simulink model "stewart_platform"  (R2013a)
settings: Solver=ode45  StartTime=0.0  StopTime=10.0  RelTol=1e-3
undefined symbols (not defined in the file): X, Y, Z
libraries: sm_lib x1374, nesl_utility x1
(part 29 of 30)

== system stewart_platform/BaseRingAssembly_1_RIGID/SwivelBearing3_1_RIGID/swivelbearingshaft_1_RIGID/Yoke_1_RIGID ==
  ReferenceFrame : sm_lib/Frames and  Transforms/Reference  Frame  BlockFunction=simmechanics.library.frames_transforms.reference_frame
  Solid : sm_lib/Body Elements/Solid  InertiaType=Custom  Mass=0.0085668099999999994  MassUnits=kg  CenterOfMass=[3.3036099999999999e-09 4.5392100000000001e-09 0.0138091]  CenterOfMassUnits=m  MomentsOfInertia=[3.6198600000000002e-07 3.7260700000000002e-07 1.1777300000000001e-07]  MomentsOfInertiaUnits=kg*m^2  ProductsOfInertia=[-1.58919e-13 -3.9281799999999999e-13 1.96468e-13]  ProductsOfInertiaUnits=kg*m^2  DensityBased=on  Density=1000  DensityUnits=kg/(m^3)  GraphicType=FromGeometry  MarkerShape=Sphere  MarkerSize=10  MarkerSizeUnits=m  GraphicVisPropType=SimpleVisualProperties  GraphicDiffuseColor=[0.594824 0.594824 0.594824]  GraphicSpecularColor=[0.5 0.5 0.5 1.0]  GraphicAmbientColor=[0.15 0.15 0.15 1.0]  GraphicEmissiveColor=[0.0 0.0 0.0 1.0]  GraphicShininess=75  GraphicOpacity=1  GeometryShape=FromFile  RectangleSize=[1 1]  RectangleSizeUnits=m  BrickDimensions=[1 1 1]  BrickDimensionUnits=m  CylinderRadius=1  CylinderRadiusUnits=m  CylinderLength=1  CylinderLengthUnits=m  SphereRadius=1  SphereRadiusUnits=m  EllipsoidRadii=[1 1 1]  EllipsoidRadiiUnits=m  ExtrusionCrossSection=[1 1; -1 1; -1 -1; 1 -1]  ExtrusionCrossSectionUnits=m  ExtrusionLength=1  ExtrusionLengthUnits=m  PolygonNumSides=3  PolygonOuterRadius=1  PolygonOuterRadiusUnits=m  ExtGeomFileName=Yoke_Default_sldprt.STL  ExtGeomFileUnits=m  RevolutionCrossSection=[1 1; 1 -1; 2 -1; 2 1]  RevolutionCrossSectionUnits=m  RevolutionExtent=Full  RevolutionAngle=180  RevolutionAngleUnits=deg  BlockFunction=simmechanics.library.body_elements.solid
  F : PMIOPort  Port=1  Side=Left
  connections:
  Solid/RConn1 -- ReferenceFrame/RConn1 -- F/RConn1

== system stewart_platform/BaseRingAssembly_1_RIGID/SwivelBearing4_1_RIGID/swivelbearingbase_1_RIGID/Bearing_Block_1_RIGID ==
  ReferenceFrame : sm_lib/Frames and  Transforms/Reference  Frame  BlockFunction=simmechanics.library.frames_transforms.reference_frame
  Solid : sm_lib/Body Elements/Solid  InertiaType=Custom  Mass=0.038815299999999997  MassUnits=kg  CenterOfMass=[1.2331699999999999 -2.0896699999999997e-06 -0.091549200000000011]  CenterOfMassUnits=cm  MomentsOfInertia=[0.037792699999999999 0.030256599999999998 0.030404499999999998]  MomentsOfInertiaUnits=kg*cm^2  ProductsOfInertia=[2.5125199999999998e-07 -0.0029988099999999998 -2.7532300000000001e-08]  ProductsOfInertiaUnits=kg*cm^2  DensityBased=on  Density=1000  DensityUnits=kg/(m^3)  GraphicType=FromGeometry  MarkerShape=Sphere  MarkerSize=10  MarkerSizeUnits=m  GraphicVisPropType=SimpleVisualProperties  GraphicDiffuseColor=[0.308706 0.308706 0.308706]  GraphicSpecularColor=[0.5 0.5 0.5 1.0]  GraphicAmbientColor=[0.15 0.15 0.15 1.0]  GraphicEmissiveColor=[0.0 0.0 0.0 1.0]  GraphicShininess=75  GraphicOpacity=1  GeometryShape=FromFile  RectangleSize=[1 1]  RectangleSizeUnits=m  BrickDimensions=[1 1 1]  BrickDimensionUnits=m  CylinderRadius=1  CylinderRadiusUnits=m  CylinderLength=1  CylinderLengthUnits=m  SphereRadius=1  SphereRadiusUnits=m  EllipsoidRadii=[1 1 1]  EllipsoidRadiiUnits=m  ExtrusionCrossSection=[1 1; -1 1; -1 -1; 1 -1]  ExtrusionCrossSectionUnits=m  ExtrusionLength=1  ExtrusionLengthUnits=m  PolygonNumSides=3  PolygonOuterRadius=1  PolygonOuterRadiusUnits=m  ExtGeomFileName=Bearing_Block_Default_sldprt.STL  ExtGeomFileUnits=cm  RevolutionCrossSection=[1 1; 1 -1; 2 -1; 2 1]  RevolutionCrossSectionUnits=m  RevolutionExtent=Full  RevolutionAngle=180  RevolutionAngleUnits=deg  BlockFunction=simmechanics.library.body_elements.solid
  F : PMIOPort  Port=1  Side=Left
  connections:
  Solid/RConn1 -- ReferenceFrame/RConn1 -- F/RConn1

== system stewart_platform/BaseRingAssembly_1_RIGID/SwivelBearing4_1_RIGID/swivelbearingbase_1_RIGID/Clevis_pin_A_3x6_1_RIGID ==
  ReferenceFrame : sm_lib/Frames and  Transforms/Reference  Frame  BlockFunction=simmechanics.library.frames_transforms.reference_frame
  Solid : sm_lib/Body Elements/Solid  InertiaType=Custom  Mass=0.00029381199999999996  MassUnits=kg  CenterOfMass=[0.29999999999999999 0 0]  CenterOfMassUnits=cm  MomentsOfInertia=[3.0689199999999997e-06 8.8308599999999993e-06 8.8308599999999993e-06]  MomentsOfInertiaUnits=kg*cm^2  ProductsOfInertia=[0 0 0]  ProductsOfInertiaUnits=kg*cm^2  DensityBased=on  Density=1000  DensityUnits=kg/(m^3)  GraphicType=FromGeometry  MarkerShape=Sphere  MarkerSize=10  MarkerSizeUnits=m  GraphicVisPropType=SimpleVisualProperties  GraphicDiffuseColor=[0.594824 0.594824 0.594824]  GraphicSpecularColor=[0.5 0.5 0.5 1.0]  GraphicAmbientColor=[0.15 0.15 0.15 1.0]  GraphicEmissiveColor=[0.0 0.0 0.0 1.0]  GraphicShininess=75  GraphicOpacity=1  GeometryShape=FromFile  RectangleSize=[1 1]  RectangleSizeUnits=m  BrickDimensions=[1 1 1]  BrickDimensionUnits=m  CylinderRadius=1  CylinderRadiusUnits=m  CylinderLength=1  CylinderLengthUnits=m  SphereRadius=1  SphereRadiusUnits=m  EllipsoidRadii=[1 1 1]  EllipsoidRadiiUnits=m  ExtrusionCrossSection=[1 1; -1 1; -1 -1; 1 -1]  ExtrusionCrossSectionUnits=m  ExtrusionLength=1  ExtrusionLengthUnits=m  PolygonNumSides=3  PolygonOuterRadius=1  PolygonOuterRadiusUnits=m  ExtGeomFileName=Clevis_pin_A_3x6_Default_sldprt.STL  ExtGeomFileUnits=cm  RevolutionCrossSection=[1 1; 1 -1; 2 -1; 2 1]  RevolutionCrossSectionUnits=m  RevolutionExtent=Full  RevolutionAngle=180  RevolutionAngleUnits=deg  BlockFunction=simmechanics.library.body_elements.solid
  F : PMIOPort  Port=1  Side=Left
  connections:
  Solid/RConn1 -- ReferenceFrame/RConn1 -- F/RConn1

== system stewart_platform/BaseRingAssembly_1_RIGID/SwivelBearing4_1_RIGID/swivelbearingbase_1_RIGID/Clevis_pin_A_3x6_2_RIGID ==
  ReferenceFrame : sm_lib/Frames and  Transforms/Reference  Frame  BlockFunction=simmechanics.library.frames_transforms.reference_frame
  Solid : sm_lib/Body Elements/Solid  InertiaType=Custom  Mass=0.00029381199999999996  MassUnits=kg  CenterOfMass=[0.29999999999999999 0 0]  CenterOfMassUnits=cm  MomentsOfInertia=[3.0689199999999997e-06 8.8308599999999993e-06 8.8308599999999993e-06]  MomentsOfInertiaUnits=kg*cm^2  ProductsOfInertia=[0 0 0]  ProductsOfInertiaUnits=kg*cm^2  DensityBased=on  Density=1000  DensityUnits=kg/(m^3)  GraphicType=FromGeometry  MarkerShape=Sphere  MarkerSize=10  MarkerSizeUnits=m  GraphicVisPropType=SimpleVisualProperties  GraphicDiffuseColor=[0.594824 0.594824 0.594824]  GraphicSpecularColor=[0.5 0.5 0.5 1.0]  GraphicAmbientColor=[0.15 0.15 0.15 1.0]  GraphicEmissiveColor=[0.0 0.0 0.0 1.0]  GraphicShininess=75  GraphicOpacity=1  GeometryShape=FromFile  RectangleSize=[1 1]  RectangleSizeUnits=m  BrickDimensions=[1 1 1]  BrickDimensionUnits=m  CylinderRadius=1  CylinderRadiusUnits=m  CylinderLength=1  CylinderLengthUnits=m  SphereRadius=1  SphereRadiusUnits=m  EllipsoidRadii=[1 1 1]  EllipsoidRadiiUnits=m  ExtrusionCrossSection=[1 1; -1 1; -1 -1; 1 -1]  ExtrusionCrossSectionUnits=m  ExtrusionLength=1  ExtrusionLengthUnits=m  PolygonNumSides=3  PolygonOuterRadius=1  PolygonOuterRadiusUnits=m  ExtGeomFileName=Clevis_pin_A_3x6_Default_sldprt.STL  ExtGeomFileUnits=cm  RevolutionCrossSection=[1 1; 1 -1; 2 -1; 2 1]  RevolutionCrossSectionUnits=m  RevolutionExtent=Full  RevolutionAngle=180  RevolutionAngleUnits=deg  BlockFunction=simmechanics.library.body_elements.solid
  F : PMIOPort  Port=1  Side=Left
  connections:
  Solid/RConn1 -- ReferenceFrame/RConn1 -- F/RConn1

== system stewart_platform/BaseRingAssembly_1_RIGID/SwivelBearing4_1_RIGID/swivelbearingbase_1_RIGID/Cylinder_Head_Cap_Screw_M3x10_1_RIGID ==
  ReferenceFrame : sm_lib/Frames and  Transforms/Reference  Frame  BlockFunction=simmechanics.library.frames_transforms.reference_frame
  Solid : sm_lib/Body Elements/Solid  InertiaType=Custom  Mass=0.00086707500000000014  MassUnits=kg  CenterOfMass=[0.27793600000000002 4.4415200000000001e-05 3.1751399999999999e-07]  CenterOfMassUnits=cm  MomentsOfInertia=[1.96811e-05 0.000127587 0.000127572]  MomentsOfInertiaUnits=kg*cm^2  ProductsOfInertia=[9.9546899999999997e-10 -9.8543100000000009e-11 -1.3784599999999999e-08]  ProductsOfInertiaUnits=kg*cm^2  DensityBased=on  Density=1000  DensityUnits=kg/(m^3)  GraphicType=FromGeometry  MarkerShape=Sphere  MarkerSize=10  MarkerSizeUnits=m  GraphicVisPropType=SimpleVisualProperties  GraphicDiffuseColor=[0.722824 0.722824 0.722824]  GraphicSpecularColor=[0.5 0.5 0.5 1.0]  GraphicAmbientColor=[0.15 0.15 0.15 1.0]  GraphicEmissiveColor=[0.0 0.0 0.0 1.0]  GraphicShininess=75  GraphicOpacity=1  GeometryShape=FromFile  RectangleSize=[1 1]  RectangleSizeUnits=m  BrickDimensions=[1 1 1]  BrickDimensionUnits=m  CylinderRadius=1  CylinderRadiusUnits=m  CylinderLength=1  CylinderLengthUnits=m  SphereRadius=1  SphereRadiusUnits=m  EllipsoidRadii=[1 1 1]  EllipsoidRadiiUnits=m  ExtrusionCrossSection=[1 1; -1 1; -1 -1; 1 -1]  ExtrusionCrossSectionUnits=m  ExtrusionLength=1  ExtrusionLengthUnits=m  PolygonNumSides=3  PolygonOuterRadius=1  PolygonOuterRadiusUnits=m  ExtGeomFileName=Cylinder_Head_Cap_Screw_M3x10_Default_sldprt.STL  ExtGeomFileUnits=cm  RevolutionCrossSection=[1 1; 1 -1; 2 -1; 2 1]  RevolutionCrossSectionUnits=m  RevolutionExtent=Full  RevolutionAngle=180  RevolutionAngleUnits=deg  BlockFunction=simmechanics.library.body_elements.solid
  F : PMIOPort  Port=1  Side=Left
  connections:
  Solid/RConn1 -- ReferenceFrame/RConn1 -- F/RConn1

== system stewart_platform/BaseRingAssembly_1_RIGID/SwivelBearing4_1_RIGID/swivelbearingbase_1_RIGID/Cylinder_Head_Cap_Screw_M3x10_2_RIGID ==
  ReferenceFrame : sm_lib/Frames and  Transforms/Reference  Frame  BlockFunction=simmechanics.library.frames_transforms.reference_frame
  Solid : sm_lib/Body Elements/Solid  InertiaType=Custom  Mass=0.00086707500000000014  MassUnits=kg  CenterOfMass=[0.27793600000000002 4.4415200000000001e-05 3.1751399999999999e-07]  CenterOfMassUnits=cm  MomentsOfInertia=[1.96811e-05 0.000127587 0.000127572]  MomentsOfInertiaUnits=kg*cm^2  ProductsOfInertia=[9.9546899999999997e-10 -9.8543100000000009e-11 -1.3784599999999999e-08]  ProductsOfInertiaUnits=kg*cm^2  DensityBased=on  Density=1000  DensityUnits=kg/(m^3)  GraphicType=FromGeometry  MarkerShape=Sphere  MarkerSize=10  MarkerSizeUnits=m  GraphicVisPropType=SimpleVisualProperties  GraphicDiffuseColor=[0.722824 0.722824 0.722824]  GraphicSpecularColor=[0.5 0.5 0.5 1.0]  GraphicAmbientColor=[0.15 0.15 0.15 1.0]  GraphicEmissiveColor=[0.0 0.0 0.0 1.0]  GraphicShininess=75  GraphicOpacity=1  GeometryShape=FromFile  RectangleSize=[1 1]  RectangleSizeUnits=m  BrickDimensions=[1 1 1]  BrickDimensionUnits=m  CylinderRadius=1  CylinderRadiusUnits=m  CylinderLength=1  CylinderLengthUnits=m  SphereRadius=1  SphereRadiusUnits=m  EllipsoidRadii=[1 1 1]  EllipsoidRadiiUnits=m  ExtrusionCrossSection=[1 1; -1 1; -1 -1; 1 -1]  ExtrusionCrossSectionUnits=m  ExtrusionLength=1  ExtrusionLengthUnits=m  PolygonNumSides=3  PolygonOuterRadius=1  PolygonOuterRadiusUnits=m  ExtGeomFileName=Cylinder_Head_Cap_Screw_M3x10_Default_sldprt.STL  ExtGeomFileUnits=cm  RevolutionCrossSection=[1 1; 1 -1; 2 -1; 2 1]  RevolutionCrossSectionUnits=m  RevolutionExtent=Full  RevolutionAngle=180  RevolutionAngleUnits=deg  BlockFunction=simmechanics.library.body_elements.solid
  F : PMIOPort  Port=1  Side=Left
  connections:
  Solid/RConn1 -- ReferenceFrame/RConn1 -- F/RConn1

== system stewart_platform/BaseRingAssembly_1_RIGID/SwivelBearing4_1_RIGID/swivelbearingbase_1_RIGID/MPB_C345MB_1_RIGID ==
  ReferenceFrame : sm_lib/Frames and  Transforms/Reference  Frame  BlockFunction=simmechanics.library.frames_transforms.reference_frame
  Solid : sm_lib/Body Elements/Solid  InertiaType=Custom  Mass=0.0062849100000000003  MassUnits=kg  CenterOfMass=[-0.00467958 0.00015178199999999999 0]  CenterOfMassUnits=cm  MomentsOfInertia=[0.0022913899999999999 0.0012611399999999998 0.0012599700000000002]  MomentsOfInertiaUnits=kg*cm^2  ProductsOfInertia=[0 8.7957900000000007e-09 4.4951200000000001e-09]  ProductsOfInertiaUnits=kg*cm^2  DensityBased=on  Density=1000  DensityUnits=kg/(m^3)  GraphicType=FromGeometry  MarkerShape=Sphere  MarkerSize=10  MarkerSizeUnits=m  GraphicVisPropType=SimpleVisualProperties  GraphicDiffuseColor=[0.722824 0.722824 0.722824]  GraphicSpecularColor=[0.5 0.5 0.5 1.0]  GraphicAmbientColor=[0.15 0.15 0.15 1.0]  GraphicEmissiveColor=[0.0 0.0 0.0 1.0]  GraphicShininess=75  GraphicOpacity=1  GeometryShape=FromFile  RectangleSize=[1 1]  RectangleSizeUnits=m  BrickDimensions=[1 1 1]  BrickDimensionUnits=m  CylinderRadius=1  CylinderRadiusUnits=m  CylinderLength=1  CylinderLengthUnits=m  SphereRadius=1  SphereRadiusUnits=m  EllipsoidRadii=[1 1 1]  EllipsoidRadiiUnits=m  ExtrusionCrossSection=[1 1; -1 1; -1 -1; 1 -1]  ExtrusionCrossSectionUnits=m  ExtrusionLength=1  ExtrusionLengthUnits=m  PolygonNumSides=3  PolygonOuterRadius=1  PolygonOuterRadiusUnits=m  ExtGeomFileName=MPB_C345MB_Default_sldprt.STL  ExtGeomFileUnits=cm  RevolutionCrossSection=[1 1; 1 -1; 2 -1; 2 1]  RevolutionCrossSectionUnits=m  RevolutionExtent=Full  RevolutionAngle=180  RevolutionAngleUnits=deg  BlockFunction=simmechanics.library.body_elements.solid
  F : PMIOPort  Port=1  Side=Left
  connections:
  Solid/RConn1 -- ReferenceFrame/RConn1 -- F/RConn1

== system stewart_platform/BaseRingAssembly_1_RIGID/SwivelBearing4_1_RIGID/swivelbearingbase_1_RIGID/MPB_C345MB_2_RIGID ==
  ReferenceFrame : sm_lib/Frames and  Transforms/Reference  Frame  BlockFunction=simmechanics.library.frames_transforms.reference_frame
  Solid : sm_lib/Body Elements/Solid  InertiaType=Custom  Mass=0.0062849100000000003  MassUnits=kg  CenterOfMass=[-0.00467958 0.00015178199999999999 0]  CenterOfMassUnits=cm  MomentsOfInertia=[0.0022913899999999999 0.0012611399999999998 0.0012599700000000002]  MomentsOfInertiaUnits=kg*cm^2  ProductsOfInertia=[0 8.7957900000000007e-09 4.4951200000000001e-09]  ProductsOfInertiaUnits=kg*cm^2  DensityBased=on  Density=1000  DensityUnits=kg/(m^3)  GraphicType=FromGeometry  MarkerShape=Sphere  MarkerSize=10  MarkerSizeUnits=m  GraphicVisPropType=SimpleVisualProperties  GraphicDiffuseColor=[0.722824 0.722824 0.722824]  GraphicSpecularColor=[0.5 0.5 0.5 1.0]  GraphicAmbientColor=[0.15 0.15 0.15 1.0]  GraphicEmissiveColor=[0.0 0.0 0.0 1.0]  GraphicShininess=75  GraphicOpacity=1  GeometryShape=FromFile  RectangleSize=[1 1]  RectangleSizeUnits=m  BrickDimensions=[1 1 1]  BrickDimensionUnits=m  CylinderRadius=1  CylinderRadiusUnits=m  CylinderLength=1  CylinderLengthUnits=m  SphereRadius=1  SphereRadiusUnits=m  EllipsoidRadii=[1 1 1]  EllipsoidRadiiUnits=m  ExtrusionCrossSection=[1 1; -1 1; -1 -1; 1 -1]  ExtrusionCrossSectionUnits=m  ExtrusionLength=1  ExtrusionLengthUnits=m  PolygonNumSides=3  PolygonOuterRadius=1  PolygonOuterRadiusUnits=m  ExtGeomFileName=MPB_C345MB_Default_sldprt.STL  ExtGeomFileUnits=cm  RevolutionCrossSection=[1 1; 1 -1; 2 -1; 2 1]  RevolutionCrossSectionUnits=m  RevolutionExtent=Full  RevolutionAngle=180  RevolutionAngleUnits=deg  BlockFunction=simmechanics.library.body_elements.solid
  F : PMIOPort  Port=1  Side=Left
  connections:
  Solid/RConn1 -- ReferenceFrame/RConn1 -- F/RConn1

== system stewart_platform/BaseRingAssembly_1_RIGID/SwivelBearing4_1_RIGID/swivelbearingshaft_1_RIGID/Hex_Nut_M5_1_RIGID ==
  ReferenceFrame : sm_lib/Frames and  Transforms/Reference  Frame  BlockFunction=simmechanics.library.frames_transforms.reference_frame
  Solid : sm_lib/Body Elements/Solid  InertiaType=Custom  Mass=0.0014621200000000001  MassUnits=kg  CenterOfMass=[0.23500000000000001 8.4057099999999999e-13 -1.6260300000000001e-12]  CenterOfMassUnits=cm  MomentsOfInertia=[0.00015881600000000002 0.000103959 0.00010395999999999999]  MomentsOfInertiaUnits=kg*cm^2  ProductsOfInertia=[-1.13877e-10 -2.0700200000000003e-10 0]  ProductsOfInertiaUnits=kg*cm^2  DensityBased=on  Density=1000  DensityUnits=kg/(m^3)  GraphicType=FromGeometry  MarkerShape=Sphere  MarkerSize=10  MarkerSizeUnits=m  GraphicVisPropType=SimpleVisualProperties  GraphicDiffuseColor=[0.594824 0.594824 0.594824]  GraphicSpecularColor=[0.5 0.5 0.5 1.0]  GraphicAmbientColor=[0.15 0.15 0.15 1.0]  GraphicEmissiveColor=[0.0 0.0 0.0 1.0]  GraphicShininess=75  GraphicOpacity=1  GeometryShape=FromFile  RectangleSize=[1 1]  RectangleSizeUnits=m  BrickDimensions=[1 1 1]  BrickDimensionUnits=m  CylinderRadius=1  CylinderRadiusUnits=m  CylinderLength=1  CylinderLengthUnits=m  SphereRadius=1  SphereRadiusUnits=m  EllipsoidRadii=[1 1 1]  EllipsoidRadiiUnits=m  ExtrusionCrossSection=[1 1; -1 1; -1 -1; 1 -1]  ExtrusionCrossSectionUnits=m  ExtrusionLength=1  ExtrusionLengthUnits=m  PolygonNumSides=3  PolygonOuterRadius=1  PolygonOuterRadiusUnits=m  ExtGeomFileName=Hex_Nut_M5_Default_sldprt.STL  ExtGeomFileUnits=cm  RevolutionCrossSection=[1 1; 1 -1; 2 -1; 2 1]  RevolutionCrossSectionUnits=m  RevolutionExtent=Full  RevolutionAngle=180  RevolutionAngleUnits=deg  BlockFunction=simmechanics.library.body_elements.solid
  F : PMIOPort  Port=1  Side=Left
  connections:
  Solid/RConn1 -- ReferenceFrame/RConn1 -- F/RConn1

== system stewart_platform/BaseRingAssembly_1_RIGID/SwivelBearing4_1_RIGID/swivelbearingshaft_1_RIGID/Threaded_Shaft_1_RIGID ==
  ReferenceFrame : sm_lib/Frames and  Transforms/Reference  Frame  BlockFunction=simmechanics.library.frames_transforms.reference_frame
  Solid : sm_lib/Body Elements/Solid  InertiaType=Custom  Mass=0.006728679999999999  MassUnits=kg  CenterOfMass=[0 -1.6645400000000003e-08 2.24966]  CenterOfMassUnits=cm  MomentsOfInertia=[0.011498500000000002 0.011501300000000001 0.00020671399999999999]  MomentsOfInertiaUnits=kg*cm^2  ProductsOfInertia=[-1.35425e-10 0 0]  ProductsOfInertiaUnits=kg*cm^2  DensityBased=on  Density=1000  DensityUnits=kg/(m^3)  GraphicType=FromGeometry  MarkerShape=Sphere  MarkerSize=10  MarkerSizeUnits=m  GraphicVisPropType=SimpleVisualProperties  GraphicDiffuseColor=[0.594824 0.594824 0.594824]  GraphicSpecularColor=[0.5 0.5 0.5 1.0]  GraphicAmbientColor=[0.15 0.15 0.15 1.0]  GraphicEmissiveColor=[0.0 0.0 0.0 1.0]  GraphicShininess=75  GraphicOpacity=1  GeometryShape=FromFile  RectangleSize=[1 1]  RectangleSizeUnits=m  BrickDimensions=[1 1 1]  BrickDimensionUnits=m  CylinderRadius=1  CylinderRadiusUnits=m  CylinderLength=1  CylinderLengthUnits=m  SphereRadius=1  SphereRadiusUnits=m  EllipsoidRadii=[1 1 1]  EllipsoidRadiiUnits=m  ExtrusionCrossSection=[1 1; -1 1; -1 -1; 1 -1]  ExtrusionCrossSectionUnits=m  ExtrusionLength=1  ExtrusionLengthUnits=m  PolygonNumSides=3  PolygonOuterRadius=1  PolygonOuterRadiusUnits=m  ExtGeomFileName=Threaded_Shaft_Default_sldprt.STL  ExtGeomFileUnits=cm  RevolutionCrossSection=[1 1; 1 -1; 2 -1; 2 1]  RevolutionCrossSectionUnits=m  RevolutionExtent=Full  RevolutionAngle=180  RevolutionAngleUnits=deg  BlockFunction=simmechanics.library.body_elements.solid
  F : PMIOPort  Port=1  Side=Left
  connections:
  Solid/RConn1 -- ReferenceFrame/RConn1 -- F/RConn1

== system stewart_platform/BaseRingAssembly_1_RIGID/SwivelBearing4_1_RIGID/swivelbearingshaft_1_RIGID/Yoke_1_RIGID ==
  ReferenceFrame : sm_lib/Frames and  Transforms/Reference  Frame  BlockFunction=simmechanics.library.frames_transforms.reference_frame
  Solid : sm_lib/Body Elements/Solid  InertiaType=Custom  Mass=0.0085668099999999994  MassUnits=kg  CenterOfMass=[3.3036099999999999e-09 4.5392100000000001e-09 0.0138091]  CenterOfMassUnits=m  MomentsOfInertia=[3.6198600000000002e-07 3.7260700000000002e-07 1.1777300000000001e-07]  MomentsOfInertiaUnits=kg*m^2  ProductsOfInertia=[-1.58919e-13 -3.9281799999999999e-13 1.96468e-13]  ProductsOfInertiaUnits=kg*m^2  DensityBased=on  Density=1000  DensityUnits=kg/(m^3)  GraphicType=FromGeometry  MarkerShape=Sphere  MarkerSize=10  MarkerSizeUnits=m  GraphicVisPropType=SimpleVisualProperties  GraphicDiffuseColor=[0.594824 0.594824 0.594824]  GraphicSpecularColor=[0.5 0.5 0.5 1.0]  GraphicAmbientColor=[0.15 0.15 0.15 1.0]  GraphicEmissiveColor=[0.0 0.0 0.0 1.0]  GraphicShininess=75  GraphicOpacity=1  GeometryShape=FromFile  RectangleSize=[1 1]  RectangleSizeUnits=m  BrickDimensions=[1 1 1]  BrickDimensionUnits=m  CylinderRadius=1  CylinderRadiusUnits=m  CylinderLength=1  CylinderLengthUnits=m  SphereRadius=1  SphereRadiusUnits=m  EllipsoidRadii=[1 1 1]  EllipsoidRadiiUnits=m  ExtrusionCrossSection=[1 1; -1 1; -1 -1; 1 -1]  ExtrusionCrossSectionUnits=m  ExtrusionLength=1  ExtrusionLengthUnits=m  PolygonNumSides=3  PolygonOuterRadius=1  PolygonOuterRadiusUnits=m  ExtGeomFileName=Yoke_Default_sldprt.STL  ExtGeomFileUnits=m  RevolutionCrossSection=[1 1; 1 -1; 2 -1; 2 1]  RevolutionCrossSectionUnits=m  RevolutionExtent=Full  RevolutionAngle=180  RevolutionAngleUnits=deg  BlockFunction=simmechanics.library.body_elements.solid
  F : PMIOPort  Port=1  Side=Left
  connections:
  Solid/RConn1 -- ReferenceFrame/RConn1 -- F/RConn1

== system stewart_platform/BaseRingAssembly_1_RIGID/SwivelBearing5_1_RIGID/swivelbearingbase_1_RIGID/Bearing_Block_1_RIGID ==
  ReferenceFrame : sm_lib/Frames and  Transforms/Reference  Frame  BlockFunction=simmechanics.library.frames_transforms.reference_frame
  Solid : sm_lib/Body Elements/Solid  InertiaType=Custom  Mass=0.038815299999999997  MassUnits=kg  CenterOfMass=[1.2331699999999999 -2.0896699999999997e-06 -0.091549200000000011]  CenterOfMassUnits=cm  MomentsOfInertia=[0.037792699999999999 0.030256599999999998 0.030404499999999998]  MomentsOfInertiaUnits=kg*cm^2  ProductsOfInertia=[2.5125199999999998e-07 -0.0029988099999999998 -2.7532300000000001e-08]  ProductsOfInertiaUnits=kg*cm^2  DensityBased=on  Density=1000  DensityUnits=kg/(m^3)  GraphicType=FromGeometry  MarkerShape=Sphere  MarkerSize=10  MarkerSizeUnits=m  GraphicVisPropType=SimpleVisualProperties  GraphicDiffuseColor=[0.308706 0.308706 0.308706]  GraphicSpecularColor=[0.5 0.5 0.5 1.0]  GraphicAmbientColor=[0.15 0.15 0.15 1.0]  GraphicEmissiveColor=[0.0 0.0 0.0 1.0]  GraphicShininess=75  GraphicOpacity=1  GeometryShape=FromFile  RectangleSize=[1 1]  RectangleSizeUnits=m  BrickDimensions=[1 1 1]  BrickDimensionUnits=m  CylinderRadius=1  CylinderRadiusUnits=m  CylinderLength=1  CylinderLengthUnits=m  SphereRadius=1  SphereRadiusUnits=m  EllipsoidRadii=[1 1 1]  EllipsoidRadiiUnits=m  ExtrusionCrossSection=[1 1; -1 1; -1 -1; 1 -1]  ExtrusionCrossSectionUnits=m  ExtrusionLength=1  ExtrusionLengthUnits=m  PolygonNumSides=3  PolygonOuterRadius=1  PolygonOuterRadiusUnits=m  ExtGeomFileName=Bearing_Block_Default_sldprt.STL  ExtGeomFileUnits=cm  RevolutionCrossSection=[1 1; 1 -1; 2 -1; 2 1]  RevolutionCrossSectionUnits=m  RevolutionExtent=Full  RevolutionAngle=180  RevolutionAngleUnits=deg  BlockFunction=simmechanics.library.body_elements.solid
  F : PMIOPort  Port=1  Side=Left
  connections:
  Solid/RConn1 -- ReferenceFrame/RConn1 -- F/RConn1

== system stewart_platform/BaseRingAssembly_1_RIGID/SwivelBearing5_1_RIGID/swivelbearingbase_1_RIGID/Clevis_pin_A_3x6_1_RIGID ==
  ReferenceFrame : sm_lib/Frames and  Transforms/Reference  Frame  BlockFunction=simmechanics.library.frames_transforms.reference_frame
  Solid : sm_lib/Body Elements/Solid  InertiaType=Custom  Mass=0.00029381199999999996  MassUnits=kg  CenterOfMass=[0.29999999999999999 0 0]  CenterOfMassUnits=cm  MomentsOfInertia=[3.0689199999999997e-06 8.8308599999999993e-06 8.8308599999999993e-06]  MomentsOfInertiaUnits=kg*cm^2  ProductsOfInertia=[0 0 0]  ProductsOfInertiaUnits=kg*cm^2  DensityBased=on  Density=1000  DensityUnits=kg/(m^3)  GraphicType=FromGeometry  MarkerShape=Sphere  MarkerSize=10  MarkerSizeUnits=m  GraphicVisPropType=SimpleVisualProperties  GraphicDiffuseColor=[0.594824 0.594824 0.594824]  GraphicSpecularColor=[0.5 0.5 0.5 1.0]  GraphicAmbientColor=[0.15 0.15 0.15 1.0]  GraphicEmissiveColor=[0.0 0.0 0.0 1.0]  GraphicShininess=75  GraphicOpacity=1  GeometryShape=FromFile  RectangleSize=[1 1]  RectangleSizeUnits=m  BrickDimensions=[1 1 1]  BrickDimensionUnits=m  CylinderRadius=1  CylinderRadiusUnits=m  CylinderLength=1  CylinderLengthUnits=m  SphereRadius=1  SphereRadiusUnits=m  EllipsoidRadii=[1 1 1]  EllipsoidRadiiUnits=m  ExtrusionCrossSection=[1 1; -1 1; -1 -1; 1 -1]  ExtrusionCrossSectionUnits=m  ExtrusionLength=1  ExtrusionLengthUnits=m  PolygonNumSides=3  PolygonOuterRadius=1  PolygonOuterRadiusUnits=m  ExtGeomFileName=Clevis_pin_A_3x6_Default_sldprt.STL  ExtGeomFileUnits=cm  RevolutionCrossSection=[1 1; 1 -1; 2 -1; 2 1]  RevolutionCrossSectionUnits=m  RevolutionExtent=Full  RevolutionAngle=180  RevolutionAngleUnits=deg  BlockFunction=simmechanics.library.body_elements.solid
  F : PMIOPort  Port=1  Side=Left
  connections:
  Solid/RConn1 -- ReferenceFrame/RConn1 -- F/RConn1

== system stewart_platform/BaseRingAssembly_1_RIGID/SwivelBearing5_1_RIGID/swivelbearingbase_1_RIGID/Clevis_pin_A_3x6_2_RIGID ==
  ReferenceFrame : sm_lib/Frames and  Transforms/Reference  Frame  BlockFunction=simmechanics.library.frames_transforms.reference_frame
  Solid : sm_lib/Body Elements/Solid  InertiaType=Custom  Mass=0.00029381199999999996  MassUnits=kg  CenterOfMass=[0.29999999999999999 0 0]  CenterOfMassUnits=cm  MomentsOfInertia=[3.0689199999999997e-06 8.8308599999999993e-06 8.8308599999999993e-06]  MomentsOfInertiaUnits=kg*cm^2  ProductsOfInertia=[0 0 0]  ProductsOfInertiaUnits=kg*cm^2  DensityBased=on  Density=1000  DensityUnits=kg/(m^3)  GraphicType=FromGeometry  MarkerShape=Sphere  MarkerSize=10  MarkerSizeUnits=m  GraphicVisPropType=SimpleVisualProperties  GraphicDiffuseColor=[0.594824 0.594824 0.594824]  GraphicSpecularColor=[0.5 0.5 0.5 1.0]  GraphicAmbientColor=[0.15 0.15 0.15 1.0]  GraphicEmissiveColor=[0.0 0.0 0.0 1.0]  GraphicShininess=75  GraphicOpacity=1  GeometryShape=FromFile  RectangleSize=[1 1]  RectangleSizeUnits=m  BrickDimensions=[1 1 1]  BrickDimensionUnits=m  CylinderRadius=1  CylinderRadiusUnits=m  CylinderLength=1  CylinderLengthUnits=m  SphereRadius=1  SphereRadiusUnits=m  EllipsoidRadii=[1 1 1]  EllipsoidRadiiUnits=m  ExtrusionCrossSection=[1 1; -1 1; -1 -1; 1 -1]  ExtrusionCrossSectionUnits=m  ExtrusionLength=1  ExtrusionLengthUnits=m  PolygonNumSides=3  PolygonOuterRadius=1  PolygonOuterRadiusUnits=m  ExtGeomFileName=Clevis_pin_A_3x6_Default_sldprt.STL  ExtGeomFileUnits=cm  RevolutionCrossSection=[1 1; 1 -1; 2 -1; 2 1]  RevolutionCrossSectionUnits=m  RevolutionExtent=Full  RevolutionAngle=180  RevolutionAngleUnits=deg  BlockFunction=simmechanics.library.body_elements.solid
  F : PMIOPort  Port=1  Side=Left
  connections:
  Solid/RConn1 -- ReferenceFrame/RConn1 -- F/RConn1

== system stewart_platform/BaseRingAssembly_1_RIGID/SwivelBearing5_1_RIGID/swivelbearingbase_1_RIGID/Cylinder_Head_Cap_Screw_M3x10_1_RIGID ==
  ReferenceFrame : sm_lib/Frames and  Transforms/Reference  Frame  BlockFunction=simmechanics.library.frames_transforms.reference_frame
  Solid : sm_lib/Body Elements/Solid  InertiaType=Custom  Mass=0.00086707500000000014  MassUnits=kg  CenterOfMass=[0.27793600000000002 4.4415200000000001e-05 3.1751399999999999e-07]  CenterOfMassUnits=cm  MomentsOfInertia=[1.96811e-05 0.000127587 0.000127572]  MomentsOfInertiaUnits=kg*cm^2  ProductsOfInertia=[9.9546899999999997e-10 -9.8543100000000009e-11 -1.3784599999999999e-08]  ProductsOfInertiaUnits=kg*cm^2  DensityBased=on  Density=1000  DensityUnits=kg/(m^3)  GraphicType=FromGeometry  MarkerShape=Sphere  MarkerSize=10  MarkerSizeUnits=m  GraphicVisPropType=SimpleVisualProperties  GraphicDiffuseColor=[0.722824 0.722824 0.722824]  GraphicSpecularColor=[0.5 0.5 0.5 1.0]  GraphicAmbientColor=[0.15 0.15 0.15 1.0]  GraphicEmissiveColor=[0.0 0.0 0.0 1.0]  GraphicShininess=75  GraphicOpacity=1  GeometryShape=FromFile  RectangleSize=[1 1]  RectangleSizeUnits=m  BrickDimensions=[1 1 1]  BrickDimensionUnits=m  CylinderRadius=1  CylinderRadiusUnits=m  CylinderLength=1  CylinderLengthUnits=m  SphereRadius=1  SphereRadiusUnits=m  EllipsoidRadii=[1 1 1]  EllipsoidRadiiUnits=m  ExtrusionCrossSection=[1 1; -1 1; -1 -1; 1 -1]  ExtrusionCrossSectionUnits=m  ExtrusionLength=1  ExtrusionLengthUnits=m  PolygonNumSides=3  PolygonOuterRadius=1  PolygonOuterRadiusUnits=m  ExtGeomFileName=Cylinder_Head_Cap_Screw_M3x10_Default_sldprt.STL  ExtGeomFileUnits=cm  RevolutionCrossSection=[1 1; 1 -1; 2 -1; 2 1]  RevolutionCrossSectionUnits=m  RevolutionExtent=Full  RevolutionAngle=180  RevolutionAngleUnits=deg  BlockFunction=simmechanics.library.body_elements.solid
  F : PMIOPort  Port=1  Side=Left
  connections:
  Solid/RConn1 -- ReferenceFrame/RConn1 -- F/RConn1

== system stewart_platform/BaseRingAssembly_1_RIGID/SwivelBearing5_1_RIGID/swivelbearingbase_1_RIGID/Cylinder_Head_Cap_Screw_M3x10_2_RIGID ==
  ReferenceFrame : sm_lib/Frames and  Transforms/Reference  Frame  BlockFunction=simmechanics.library.frames_transforms.reference_frame
  Solid : sm_lib/Body Elements/Solid  InertiaType=Custom  Mass=0.00086707500000000014  MassUnits=kg  CenterOfMass=[0.27793600000000002 4.4415200000000001e-05 3.1751399999999999e-07]  CenterOfMassUnits=cm  MomentsOfInertia=[1.96811e-05 0.000127587 0.000127572]  MomentsOfInertiaUnits=kg*cm^2  ProductsOfInertia=[9.9546899999999997e-10 -9.8543100000000009e-11 -1.3784599999999999e-08]  ProductsOfInertiaUnits=kg*cm^2  DensityBased=on  Density=1000  DensityUnits=kg/(m^3)  GraphicType=FromGeometry  MarkerShape=Sphere  MarkerSize=10  MarkerSizeUnits=m  GraphicVisPropType=SimpleVisualProperties  GraphicDiffuseColor=[0.722824 0.722824 0.722824]  GraphicSpecularColor=[0.5 0.5 0.5 1.0]  GraphicAmbientColor=[0.15 0.15 0.15 1.0]  GraphicEmissiveColor=[0.0 0.0 0.0 1.0]  GraphicShininess=75  GraphicOpacity=1  GeometryShape=FromFile  RectangleSize=[1 1]  RectangleSizeUnits=m  BrickDimensions=[1 1 1]  BrickDimensionUnits=m  CylinderRadius=1  CylinderRadiusUnits=m  CylinderLength=1  CylinderLengthUnits=m  SphereRadius=1  SphereRadiusUnits=m  EllipsoidRadii=[1 1 1]  EllipsoidRadiiUnits=m  ExtrusionCrossSection=[1 1; -1 1; -1 -1; 1 -1]  ExtrusionCrossSectionUnits=m  ExtrusionLength=1  ExtrusionLengthUnits=m  PolygonNumSides=3  PolygonOuterRadius=1  PolygonOuterRadiusUnits=m  ExtGeomFileName=Cylinder_Head_Cap_Screw_M3x10_Default_sldprt.STL  ExtGeomFileUnits=cm  RevolutionCrossSection=[1 1; 1 -1; 2 -1; 2 1]  RevolutionCrossSectionUnits=m  RevolutionExtent=Full  RevolutionAngle=180  RevolutionAngleUnits=deg  BlockFunction=simmechanics.library.body_elements.solid
  F : PMIOPort  Port=1  Side=Left
  connections:
  Solid/RConn1 -- ReferenceFrame/RConn1 -- F/RConn1

== system stewart_platform/BaseRingAssembly_1_RIGID/SwivelBearing5_1_RIGID/swivelbearingbase_1_RIGID/MPB_C345MB_1_RIGID ==
  ReferenceFrame : sm_lib/Frames and  Transforms/Reference  Frame  BlockFunction=simmechanics.library.frames_transforms.reference_frame
  Solid : sm_lib/Body Elements/Solid  InertiaType=Custom  Mass=0.0062849100000000003  MassUnits=kg  CenterOfMass=[-0.00467958 0.00015178199999999999 0]  CenterOfMassUnits=cm  MomentsOfInertia=[0.0022913899999999999 0.0012611399999999998 0.0012599700000000002]  MomentsOfInertiaUnits=kg*cm^2  ProductsOfInertia=[0 8.7957900000000007e-09 4.4951200000000001e-09]  ProductsOfInertiaUnits=kg*cm^2  DensityBased=on  Density=1000  DensityUnits=kg/(m^3)  GraphicType=FromGeometry  MarkerShape=Sphere  MarkerSize=10  MarkerSizeUnits=m  GraphicVisPropType=SimpleVisualProperties  GraphicDiffuseColor=[0.722824 0.722824 0.722824]  GraphicSpecularColor=[0.5 0.5 0.5 1.0]  GraphicAmbientColor=[0.15 0.15 0.15 1.0]  GraphicEmissiveColor=[0.0 0.0 0.0 1.0]  GraphicShininess=75  GraphicOpacity=1  GeometryShape=FromFile  RectangleSize=[1 1]  RectangleSizeUnits=m  BrickDimensions=[1 1 1]  BrickDimensionUnits=m  CylinderRadius=1  CylinderRadiusUnits=m  CylinderLength=1  CylinderLengthUnits=m  SphereRadius=1  SphereRadiusUnits=m  EllipsoidRadii=[1 1 1]  EllipsoidRadiiUnits=m  ExtrusionCrossSection=[1 1; -1 1; -1 -1; 1 -1]  ExtrusionCrossSectionUnits=m  ExtrusionLength=1  ExtrusionLengthUnits=m  PolygonNumSides=3  PolygonOuterRadius=1  PolygonOuterRadiusUnits=m  ExtGeomFileName=MPB_C345MB_Default_sldprt.STL  ExtGeomFileUnits=cm  RevolutionCrossSection=[1 1; 1 -1; 2 -1; 2 1]  RevolutionCrossSectionUnits=m  RevolutionExtent=Full  RevolutionAngle=180  RevolutionAngleUnits=deg  BlockFunction=simmechanics.library.body_elements.solid
  F : PMIOPort  Port=1  Side=Left
  connections:
  Solid/RConn1 -- ReferenceFrame/RConn1 -- F/RConn1

== system stewart_platform/BaseRingAssembly_1_RIGID/SwivelBearing5_1_RIGID/swivelbearingbase_1_RIGID/MPB_C345MB_2_RIGID ==
  ReferenceFrame : sm_lib/Frames and  Transforms/Reference  Frame  BlockFunction=simmechanics.library.frames_transforms.reference_frame
  Solid : sm_lib/Body Elements/Solid  InertiaType=Custom  Mass=0.0062849100000000003  MassUnits=kg  CenterOfMass=[-0.00467958 0.00015178199999999999 0]  CenterOfMassUnits=cm  MomentsOfInertia=[0.0022913899999999999 0.0012611399999999998 0.0012599700000000002]  MomentsOfInertiaUnits=kg*cm^2  ProductsOfInertia=[0 8.7957900000000007e-09 4.4951200000000001e-09]  ProductsOfInertiaUnits=kg*cm^2  DensityBased=on  Density=1000  DensityUnits=kg/(m^3)  GraphicType=FromGeometry  MarkerShape=Sphere  MarkerSize=10  MarkerSizeUnits=m  GraphicVisPropType=SimpleVisualProperties  GraphicDiffuseColor=[0.722824 0.722824 0.722824]  GraphicSpecularColor=[0.5 0.5 0.5 1.0]  GraphicAmbientColor=[0.15 0.15 0.15 1.0]  GraphicEmissiveColor=[0.0 0.0 0.0 1.0]  GraphicShininess=75  GraphicOpacity=1  GeometryShape=FromFile  RectangleSize=[1 1]  RectangleSizeUnits=m  BrickDimensions=[1 1 1]  BrickDimensionUnits=m  CylinderRadius=1  CylinderRadiusUnits=m  CylinderLength=1  CylinderLengthUnits=m  SphereRadius=1  SphereRadiusUnits=m  EllipsoidRadii=[1 1 1]  EllipsoidRadiiUnits=m  ExtrusionCrossSection=[1 1; -1 1; -1 -1; 1 -1]  ExtrusionCrossSectionUnits=m  ExtrusionLength=1  ExtrusionLengthUnits=m  PolygonNumSides=3  PolygonOuterRadius=1  PolygonOuterRadiusUnits=m  ExtGeomFileName=MPB_C345MB_Default_sldprt.STL  ExtGeomFileUnits=cm  RevolutionCrossSection=[1 1; 1 -1; 2 -1; 2 1]  RevolutionCrossSectionUnits=m  RevolutionExtent=Full  RevolutionAngle=180  RevolutionAngleUnits=deg  BlockFunction=simmechanics.library.body_elements.solid
  F : PMIOPort  Port=1  Side=Left
  connections:
  Solid/RConn1 -- ReferenceFrame/RConn1 -- F/RConn1

== system stewart_platform/BaseRingAssembly_1_RIGID/SwivelBearing5_1_RIGID/swivelbearingshaft_1_RIGID/Hex_Nut_M5_1_RIGID ==
  ReferenceFrame : sm_lib/Frames and  Transforms/Reference  Frame  BlockFunction=simmechanics.library.frames_transforms.reference_frame
  Solid : sm_lib/Body Elements/Solid  InertiaType=Custom  Mass=0.0014621200000000001  MassUnits=kg  CenterOfMass=[0.23500000000000001 8.4057099999999999e-13 -1.6260300000000001e-12]  CenterOfMassUnits=cm  MomentsOfInertia=[0.00015881600000000002 0.000103959 0.00010395999999999999]  MomentsOfInertiaUnits=kg*cm^2  ProductsOfInertia=[-1.13877e-10 -2.0700200000000003e-10 0]  ProductsOfInertiaUnits=kg*cm^2  DensityBased=on  Density=1000  DensityUnits=kg/(m^3)  GraphicType=FromGeometry  MarkerShape=Sphere  MarkerSize=10  MarkerSizeUnits=m  GraphicVisPropType=SimpleVisualProperties  GraphicDiffuseColor=[0.594824 0.594824 0.594824]  GraphicSpecularColor=[0.5 0.5 0.5 1.0]  GraphicAmbientColor=[0.15 0.15 0.15 1.0]  GraphicEmissiveColor=[0.0 0.0 0.0 1.0]  GraphicShininess=75  GraphicOpacity=1  GeometryShape=FromFile  RectangleSize=[1 1]  RectangleSizeUnits=m  BrickDimensions=[1 1 1]  BrickDimensionUnits=m  CylinderRadius=1  CylinderRadiusUnits=m  CylinderLength=1  CylinderLengthUnits=m  SphereRadius=1  SphereRadiusUnits=m  EllipsoidRadii=[1 1 1]  EllipsoidRadiiUnits=m  ExtrusionCrossSection=[1 1; -1 1; -1 -1; 1 -1]  ExtrusionCrossSectionUnits=m  ExtrusionLength=1  ExtrusionLengthUnits=m  PolygonNumSides=3  PolygonOuterRadius=1  PolygonOuterRadiusUnits=m  ExtGeomFileName=Hex_Nut_M5_Default_sldprt.STL  ExtGeomFileUnits=cm  RevolutionCrossSection=[1 1; 1 -1; 2 -1; 2 1]  RevolutionCrossSectionUnits=m  RevolutionExtent=Full  RevolutionAngle=180  RevolutionAngleUnits=deg  BlockFunction=simmechanics.library.body_elements.solid
  F : PMIOPort  Port=1  Side=Left
  connections:
  Solid/RConn1 -- ReferenceFrame/RConn1 -- F/RConn1

== system stewart_platform/BaseRingAssembly_1_RIGID/SwivelBearing5_1_RIGID/swivelbearingshaft_1_RIGID/Threaded_Shaft_1_RIGID ==
  ReferenceFrame : sm_lib/Frames and  Transforms/Reference  Frame  BlockFunction=simmechanics.library.frames_transforms.reference_frame
  Solid : sm_lib/Body Elements/Solid  InertiaType=Custom  Mass=0.006728679999999999  MassUnits=kg  CenterOfMass=[0 -1.6645400000000003e-08 2.24966]  CenterOfMassUnits=cm  MomentsOfInertia=[0.011498500000000002 0.011501300000000001 0.00020671399999999999]  MomentsOfInertiaUnits=kg*cm^2  ProductsOfInertia=[-1.35425e-10 0 0]  ProductsOfInertiaUnits=kg*cm^2  DensityBased=on  Density=1000  DensityUnits=kg/(m^3)  GraphicType=FromGeometry  MarkerShape=Sphere  MarkerSize=10  MarkerSizeUnits=m  GraphicVisPropType=SimpleVisualProperties  GraphicDiffuseColor=[0.594824 0.594824 0.594824]  GraphicSpecularColor=[0.5 0.5 0.5 1.0]  GraphicAmbientColor=[0.15 0.15 0.15 1.0]  GraphicEmissiveColor=[0.0 0.0 0.0 1.0]  GraphicShininess=75  GraphicOpacity=1  GeometryShape=FromFile  RectangleSize=[1 1]  RectangleSizeUnits=m  BrickDimensions=[1 1 1]  BrickDimensionUnits=m  CylinderRadius=1  CylinderRadiusUnits=m  CylinderLength=1  CylinderLengthUnits=m  SphereRadius=1  SphereRadiusUnits=m  EllipsoidRadii=[1 1 1]  EllipsoidRadiiUnits=m  ExtrusionCrossSection=[1 1; -1 1; -1 -1; 1 -1]  ExtrusionCrossSectionUnits=m  ExtrusionLength=1  ExtrusionLengthUnits=m  PolygonNumSides=3  PolygonOuterRadius=1  PolygonOuterRadiusUnits=m  ExtGeomFileName=Threaded_Shaft_Default_sldprt.STL  ExtGeomFileUnits=cm  RevolutionCrossSection=[1 1; 1 -1; 2 -1; 2 1]  RevolutionCrossSectionUnits=m  RevolutionExtent=Full  RevolutionAngle=180  RevolutionAngleUnits=deg  BlockFunction=simmechanics.library.body_elements.solid
  F : PMIOPort  Port=1  Side=Left
  connections:
  Solid/RConn1 -- ReferenceFrame/RConn1 -- F/RConn1

== system stewart_platform/BaseRingAssembly_1_RIGID/SwivelBearing5_1_RIGID/swivelbearingshaft_1_RIGID/Yoke_1_RIGID ==
  ReferenceFrame : sm_lib/Frames and  Transforms/Reference  Frame  BlockFunction=simmechanics.library.frames_transforms.reference_frame
  Solid : sm_lib/Body Elements/Solid  InertiaType=Custom  Mass=0.0085668099999999994  MassUnits=kg  CenterOfMass=[3.3036099999999999e-09 4.5392100000000001e-09 0.0138091]  CenterOfMassUnits=m  MomentsOfInertia=[3.6198600000000002e-07 3.7260700000000002e-07 1.1777300000000001e-07]  MomentsOfInertiaUnits=kg*m^2  ProductsOfInertia=[-1.58919e-13 -3.9281799999999999e-13 1.96468e-13]  ProductsOfInertiaUnits=kg*m^2  DensityBased=on  Density=1000  DensityUnits=kg/(m^3)  GraphicType=FromGeometry  MarkerShape=Sphere  MarkerSize=10  MarkerSizeUnits=m  GraphicVisPropType=SimpleVisualProperties  GraphicDiffuseColor=[0.594824 0.594824 0.594824]  GraphicSpecularColor=[0.5 0.5 0.5 1.0]  GraphicAmbientColor=[0.15 0.15 0.15 1.0]  GraphicEmissiveColor=[0.0 0.0 0.0 1.0]  GraphicShininess=75  GraphicOpacity=1  GeometryShape=FromFile  RectangleSize=[1 1]  RectangleSizeUnits=m  BrickDimensions=[1 1 1]  BrickDimensionUnits=m  CylinderRadius=1  CylinderRadiusUnits=m  CylinderLength=1  CylinderLengthUnits=m  SphereRadius=1  SphereRadiusUnits=m  EllipsoidRadii=[1 1 1]  EllipsoidRadiiUnits=m  ExtrusionCrossSection=[1 1; -1 1; -1 -1; 1 -1]  ExtrusionCrossSectionUnits=m  ExtrusionLength=1  ExtrusionLengthUnits=m  PolygonNumSides=3  PolygonOuterRadius=1  PolygonOuterRadiusUnits=m  ExtGeomFileName=Yoke_Default_sldprt.STL  ExtGeomFileUnits=m  RevolutionCrossSection=[1 1; 1 -1; 2 -1; 2 1]  RevolutionCrossSectionUnits=m  RevolutionExtent=Full  RevolutionAngle=180  RevolutionAngleUnits=deg  BlockFunction=simmechanics.library.body_elements.solid
  F : PMIOPort  Port=1  Side=Left
  connections:
  Solid/RConn1 -- ReferenceFrame/RConn1 -- F/RConn1

== system stewart_platform/BaseRingAssembly_1_RIGID/SwivelBearing6_1_RIGID/swivelbearingbase_1_RIGID/Bearing_Block_1_RIGID ==
  ReferenceFrame : sm_lib/Frames and  Transforms/Reference  Frame  BlockFunction=simmechanics.library.frames_transforms.reference_frame
  Solid : sm_lib/Body Elements/Solid  InertiaType=Custom  Mass=0.038815299999999997  MassUnits=kg  CenterOfMass=[1.2331699999999999 -2.0896699999999997e-06 -0.091549200000000011]  CenterOfMassUnits=cm  MomentsOfInertia=[0.037792699999999999 0.030256599999999998 0.030404499999999998]  MomentsOfInertiaUnits=kg*cm^2  ProductsOfInertia=[2.5125199999999998e-07 -0.0029988099999999998 -2.7532300000000001e-08]  ProductsOfInertiaUnits=kg*cm^2  DensityBased=on  Density=1000  DensityUnits=kg/(m^3)  GraphicType=FromGeometry  MarkerShape=Sphere  MarkerSize=10  MarkerSizeUnits=m  GraphicVisPropType=SimpleVisualProperties  GraphicDiffuseColor=[0.308706 0.308706 0.308706]  GraphicSpecularColor=[0.5 0.5 0.5 1.0]  GraphicAmbientColor=[0.15 0.15 0.15 1.0]  GraphicEmissiveColor=[0.0 0.0 0.0 1.0]  GraphicShininess=75  GraphicOpacity=1  GeometryShape=FromFile  RectangleSize=[1 1]  RectangleSizeUnits=m  BrickDimensions=[1 1 1]  BrickDimensionUnits=m  CylinderRadius=1  CylinderRadiusUnits=m  CylinderLength=1  CylinderLengthUnits=m  SphereRadius=1  SphereRadiusUnits=m  EllipsoidRadii=[1 1 1]  EllipsoidRadiiUnits=m  ExtrusionCrossSection=[1 1; -1 1; -1 -1; 1 -1]  ExtrusionCrossSectionUnits=m  ExtrusionLength=1  ExtrusionLengthUnits=m  PolygonNumSides=3  PolygonOuterRadius=1  PolygonOuterRadiusUnits=m  ExtGeomFileName=Bearing_Block_Default_sldprt.STL  ExtGeomFileUnits=cm  RevolutionCrossSection=[1 1; 1 -1; 2 -1; 2 1]  RevolutionCrossSectionUnits=m  RevolutionExtent=Full  RevolutionAngle=180  RevolutionAngleUnits=deg  BlockFunction=simmechanics.library.body_elements.solid
  F : PMIOPort  Port=1  Side=Left
  connections:
  Solid/RConn1 -- ReferenceFrame/RConn1 -- F/RConn1

== system stewart_platform/BaseRingAssembly_1_RIGID/SwivelBearing6_1_RIGID/swivelbearingbase_1_RIGID/Clevis_pin_A_3x6_1_RIGID ==
  ReferenceFrame : sm_lib/Frames and  Transforms/Reference  Frame  BlockFunction=simmechanics.library.frames_transforms.reference_frame
  Solid : sm_lib/Body Elements/Solid  InertiaType=Custom  Mass=0.00029381199999999996  MassUnits=kg  CenterOfMass=[0.29999999999999999 0 0]  CenterOfMassUnits=cm  MomentsOfInertia=[3.0689199999999997e-06 8.8308599999999993e-06 8.8308599999999993e-06]  MomentsOfInertiaUnits=kg*cm^2  ProductsOfInertia=[0 0 0]  ProductsOfInertiaUnits=kg*cm^2  DensityBased=on  Density=1000  DensityUnits=kg/(m^3)  GraphicType=FromGeometry  MarkerShape=Sphere  MarkerSize=10  MarkerSizeUnits=m  GraphicVisPropType=SimpleVisualProperties  GraphicDiffuseColor=[0.594824 0.594824 0.594824]  GraphicSpecularColor=[0.5 0.5 0.5 1.0]  GraphicAmbientColor=[0.15 0.15 0.15 1.0]  GraphicEmissiveColor=[0.0 0.0 0.0 1.0]  GraphicShininess=75  GraphicOpacity=1  GeometryShape=FromFile  RectangleSize=[1 1]  RectangleSizeUnits=m  BrickDimensions=[1 1 1]  BrickDimensionUnits=m  CylinderRadius=1  CylinderRadiusUnits=m  CylinderLength=1  CylinderLengthUnits=m  SphereRadius=1  SphereRadiusUnits=m  EllipsoidRadii=[1 1 1]  EllipsoidRadiiUnits=m  ExtrusionCrossSection=[1 1; -1 1; -1 -1; 1 -1]  ExtrusionCrossSectionUnits=m  ExtrusionLength=1  ExtrusionLengthUnits=m  PolygonNumSides=3  PolygonOuterRadius=1  PolygonOuterRadiusUnits=m  ExtGeomFileName=Clevis_pin_A_3x6_Default_sldprt.STL  ExtGeomFileUnits=cm  RevolutionCrossSection=[1 1; 1 -1; 2 -1; 2 1]  RevolutionCrossSectionUnits=m  RevolutionExtent=Full  RevolutionAngle=180  RevolutionAngleUnits=deg  BlockFunction=simmechanics.library.body_elements.solid
  F : PMIOPort  Port=1  Side=Left
  connections:
  Solid/RConn1 -- ReferenceFrame/RConn1 -- F/RConn1

== system stewart_platform/BaseRingAssembly_1_RIGID/SwivelBearing6_1_RIGID/swivelbearingbase_1_RIGID/Clevis_pin_A_3x6_2_RIGID ==
  ReferenceFrame : sm_lib/Frames and  Transforms/Reference  Frame  BlockFunction=simmechanics.library.frames_transforms.reference_frame
  Solid : sm_lib/Body Elements/Solid  InertiaType=Custom  Mass=0.00029381199999999996  MassUnits=kg  CenterOfMass=[0.29999999999999999 0 0]  CenterOfMassUnits=cm  MomentsOfInertia=[3.0689199999999997e-06 8.8308599999999993e-06 8.8308599999999993e-06]  MomentsOfInertiaUnits=kg*cm^2  ProductsOfInertia=[0 0 0]  ProductsOfInertiaUnits=kg*cm^2  DensityBased=on  Density=1000  DensityUnits=kg/(m^3)  GraphicType=FromGeometry  MarkerShape=Sphere  MarkerSize=10  MarkerSizeUnits=m  GraphicVisPropType=SimpleVisualProperties  GraphicDiffuseColor=[0.594824 0.594824 0.594824]  GraphicSpecularColor=[0.5 0.5 0.5 1.0]  GraphicAmbientColor=[0.15 0.15 0.15 1.0]  GraphicEmissiveColor=[0.0 0.0 0.0 1.0]  GraphicShininess=75  GraphicOpacity=1  GeometryShape=FromFile  RectangleSize=[1 1]  RectangleSizeUnits=m  BrickDimensions=[1 1 1]  BrickDimensionUnits=m  CylinderRadius=1  CylinderRadiusUnits=m  CylinderLength=1  CylinderLengthUnits=m  SphereRadius=1  SphereRadiusUnits=m  EllipsoidRadii=[1 1 1]  EllipsoidRadiiUnits=m  ExtrusionCrossSection=[1 1; -1 1; -1 -1; 1 -1]  ExtrusionCrossSectionUnits=m  ExtrusionLength=1  ExtrusionLengthUnits=m  PolygonNumSides=3  PolygonOuterRadius=1  PolygonOuterRadiusUnits=m  ExtGeomFileName=Clevis_pin_A_3x6_Default_sldprt.STL  ExtGeomFileUnits=cm  RevolutionCrossSection=[1 1; 1 -1; 2 -1; 2 1]  RevolutionCrossSectionUnits=m  RevolutionExtent=Full  RevolutionAngle=180  RevolutionAngleUnits=deg  BlockFunction=simmechanics.library.body_elements.solid
  F : PMIOPort  Port=1  Side=Left
  connections:
  Solid/RConn1 -- ReferenceFrame/RConn1 -- F/RConn1

== system stewart_platform/BaseRingAssembly_1_RIGID/SwivelBearing6_1_RIGID/swivelbearingbase_1_RIGID/Cylinder_Head_Cap_Screw_M3x10_1_RIGID ==
  ReferenceFrame : sm_lib/Frames and  Transforms/Reference  Frame  BlockFunction=simmechanics.library.frames_transforms.reference_frame
  Solid : sm_lib/Body Elements/Solid  InertiaType=Custom  Mass=0.00086707500000000014  MassUnits=kg  CenterOfMass=[0.27793600000000002 4.4415200000000001e-05 3.1751399999999999e-07]  CenterOfMassUnits=cm  MomentsOfInertia=[1.96811e-05 0.000127587 0.000127572]  MomentsOfInertiaUnits=kg*cm^2  ProductsOfInertia=[9.9546899999999997e-10 -9.8543100000000009e-11 -1.3784599999999999e-08]  ProductsOfInertiaUnits=kg*cm^2  DensityBased=on  Density=1000  DensityUnits=kg/(m^3)  GraphicType=FromGeometry  MarkerShape=Sphere  MarkerSize=10  MarkerSizeUnits=m  GraphicVisPropType=SimpleVisualProperties  GraphicDiffuseColor=[0.722824 0.722824 0.722824]  GraphicSpecularColor=[0.5 0.5 0.5 1.0]  GraphicAmbientColor=[0.15 0.15 0.15 1.0]  GraphicEmissiveColor=[0.0 0.0 0.0 1.0]  GraphicShininess=75  GraphicOpacity=1  GeometryShape=FromFile  RectangleSize=[1 1]  RectangleSizeUnits=m  BrickDimensions=[1 1 1]  BrickDimensionUnits=m  CylinderRadius=1  CylinderRadiusUnits=m  CylinderLength=1  CylinderLengthUnits=m  SphereRadius=1  SphereRadiusUnits=m  EllipsoidRadii=[1 1 1]  EllipsoidRadiiUnits=m  ExtrusionCrossSection=[1 1; -1 1; -1 -1; 1 -1]  ExtrusionCrossSectionUnits=m  ExtrusionLength=1  ExtrusionLengthUnits=m  PolygonNumSides=3  PolygonOuterRadius=1  PolygonOuterRadiusUnits=m  ExtGeomFileName=Cylinder_Head_Cap_Screw_M3x10_Default_sldprt.STL  ExtGeomFileUnits=cm  RevolutionCrossSection=[1 1; 1 -1; 2 -1; 2 1]  RevolutionCrossSectionUnits=m  RevolutionExtent=Full  RevolutionAngle=180  RevolutionAngleUnits=deg  BlockFunction=simmechanics.library.body_elements.solid
  F : PMIOPort  Port=1  Side=Left
  connections:
  Solid/RConn1 -- ReferenceFrame/RConn1 -- F/RConn1

== system stewart_platform/BaseRingAssembly_1_RIGID/SwivelBearing6_1_RIGID/swivelbearingbase_1_RIGID/Cylinder_Head_Cap_Screw_M3x10_2_RIGID ==
  ReferenceFrame : sm_lib/Frames and  Transforms/Reference  Frame  BlockFunction=simmechanics.library.frames_transforms.reference_frame
  Solid : sm_lib/Body Elements/Solid  InertiaType=Custom  Mass=0.00086707500000000014  MassUnits=kg  CenterOfMass=[0.27793600000000002 4.4415200000000001e-05 3.1751399999999999e-07]  CenterOfMassUnits=cm  MomentsOfInertia=[1.96811e-05 0.000127587 0.000127572]  MomentsOfInertiaUnits=kg*cm^2  ProductsOfInertia=[9.9546899999999997e-10 -9.8543100000000009e-11 -1.3784599999999999e-08]  ProductsOfInertiaUnits=kg*cm^2  DensityBased=on  Density=1000  DensityUnits=kg/(m^3)  GraphicType=FromGeometry  MarkerShape=Sphere  MarkerSize=10  MarkerSizeUnits=m  GraphicVisPropType=SimpleVisualProperties  GraphicDiffuseColor=[0.722824 0.722824 0.722824]  GraphicSpecularColor=[0.5 0.5 0.5 1.0]  GraphicAmbientColor=[0.15 0.15 0.15 1.0]  GraphicEmissiveColor=[0.0 0.0 0.0 1.0]  GraphicShininess=75  GraphicOpacity=1  GeometryShape=FromFile  RectangleSize=[1 1]  RectangleSizeUnits=m  BrickDimensions=[1 1 1]  BrickDimensionUnits=m  CylinderRadius=1  CylinderRadiusUnits=m  CylinderLength=1  CylinderLengthUnits=m  SphereRadius=1  SphereRadiusUnits=m  EllipsoidRadii=[1 1 1]  EllipsoidRadiiUnits=m  ExtrusionCrossSection=[1 1; -1 1; -1 -1; 1 -1]  ExtrusionCrossSectionUnits=m  ExtrusionLength=1  ExtrusionLengthUnits=m  PolygonNumSides=3  PolygonOuterRadius=1  PolygonOuterRadiusUnits=m  ExtGeomFileName=Cylinder_Head_Cap_Screw_M3x10_Default_sldprt.STL  ExtGeomFileUnits=cm  RevolutionCrossSection=[1 1; 1 -1; 2 -1; 2 1]  RevolutionCrossSectionUnits=m  RevolutionExtent=Full  RevolutionAngle=180  RevolutionAngleUnits=deg  BlockFunction=simmechanics.library.body_elements.solid
  F : PMIOPort  Port=1  Side=Left
  connections:
  Solid/RConn1 -- ReferenceFrame/RConn1 -- F/RConn1
